simulink subsystem "LedsBattery"  (R2022b)
settings: Solver=VariableStepAuto  StartTime=0.0  StopTime=10.0  RelTol=1e-3
libraries: arduinolib x2
settings Model: Creator=dar.io  LastModifiedBy=Usuario

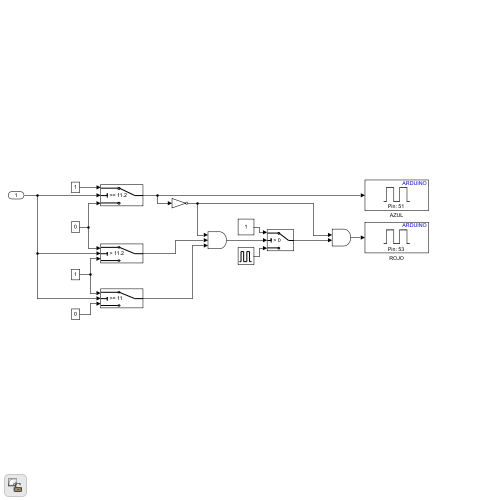
[thumbnail: Simulink's stored preview of the top-level diagram]
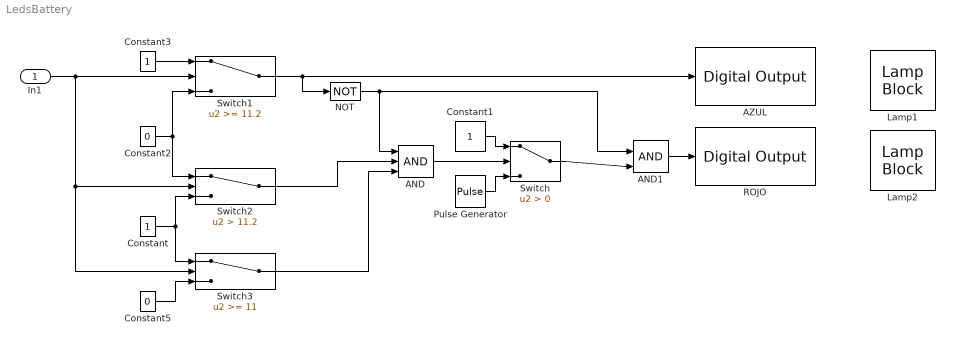
== system LedsBattery ==
  In1 : Inport  OutDataTypeStr=double
  AND : Logic  Inputs=3  IconShape=distinctive  AllPortsSameDT=off  OutDataTypeStr=boolean
  AND1 : Logic  IconShape=distinctive  AllPortsSameDT=off  OutDataTypeStr=boolean
  AZUL : arduinolib/Digital Output  pinNumber=51  Direction=output  blockPlatform=arduino
  Constant : Constant
  Constant1 : Constant
  Constant2 : Constant  Value=0
  Constant3 : Constant
  Constant5 : Constant  Value=0
  Lamp1 : LampBlock  LabelPosition=Hide
  Lamp2 : LampBlock  LabelPosition=Hide
  NOT : Logic  Operator=NOT  IconShape=distinctive  AllPortsSameDT=off  OutDataTypeStr=boolean
  Pulse Generator : DiscretePulseGenerator  PulseType=Time based  Period=1  PulseWidth=50
  ROJO : arduinolib/Digital Output  pinNumber=53  Direction=output  blockPlatform=arduino
  Switch : Switch  Criteria=u2 > Threshold  SaturateOnIntegerOverflow=off  InputSameDT=off
  Switch1 : Switch  Threshold=11.2  OutDataTypeStr=double  SaturateOnIntegerOverflow=off  InputSameDT=off
  Switch2 : Switch  Criteria=u2 > Threshold  Threshold=11.2  OutDataTypeStr=double  SaturateOnIntegerOverflow=off  InputSameDT=off
  Switch3 : Switch  Threshold=11  OutDataTypeStr=double  SaturateOnIntegerOverflow=off  InputSameDT=off
  wires:
  Constant5/1 -> Switch3/3
  Constant3/1 -> Switch1/1
  Constant2/1 -> Switch1/3, Switch2/1
  Constant/1 -> Switch3/1, Switch2/3
  Switch/1 -> AND1/2
  AND/1 -> Switch/2
  Pulse Generator/1 -> Switch/3
  In1/1 -> Switch3/2, Switch2/2, Switch1/2
  Switch3/1 -> AND/3
  Constant1/1 -> Switch/1
  NOT/1 -> AND/1, AND1/1
  AND1/1 -> ROJO/1
  Switch2/1 -> AND/2
  Switch1/1 -> NOT/1, AZUL/1
